simulink model "N3Z_tonetest14b"  (R2014b)
settings: Solver=ode3  SolverMode=SingleTasking  StartTime=0.0  StopTime=1e-4  FixedStep=fpgaclk  RelTol=1e-3
PreLoadFcn:
  | %fpgaclk=1/32.768e6
  | fpgaclk=1/49.162e6
  | 
  | SerialData=[1,zeros(1,11),1,0,0,1]
  | load ../N3workingG/window
  | win=win';  %Go back to using flatter and wider windowed sync function
  | %load ../N3workingG/hanning    %use Hahn window
  | 
  | load ../N3workingG/PREemphasis   %For pre-empasis and deemphasis FIRs
  | 
  | %LUT3=xls2LUT2('../IQI_Qdemod.xls'); LUT3
  | load ../N3workingG/LUT3
  | load ../N3workingG/FIRiq2
  | % xls2LUT
  | 
  | GetProgFiles
  | 
  | PinAssignments    %Get Pin references for TE0722
  | 
  | 
  | 
  | 
  | 
  | %LCD
  | LCDdata=[LCD_D7,LCD_D6,LCD_D5,LCD_D4,LCD_D3,LCD_D2,LCD_D1,LCD_D0] %Note MSB...LSB!
  | LCDctrl=[LCD_E,LCD_RW,LCD_RS];
  | 
  | %for RS232 on pins 3 and 5 of USBB
  | 
  | %BT chip connections for WT12
  | 
  | RX_BT=RXD
  | TX_BT=TXD
  | 
  | RST_BB=RES
  | 
  | %PCMC=PCMC
  | %PCMS=PCMS
  | %PCMI=PCMI
  | %PCMO=PCMO
  | 
  | %Aliases:
  | SRDBT=PCMI
  | STDBT=PCMO
  | SCLK_BT=PCMC
  | SFS_BT=PCMS
  | 
  | %ADC control
  | 
  | %SDOA=SDOA
  | %SDOB=SDOB
  | %SCK=SCK
  | CONV=Csbar
  | CAL=Cal
  | 
  | ADC_G=[ADC_G3,ADC_G2,ADC_G1,ADC_G0]
  | %PD settings hard coded now
  | 
  | %%%%%%
  | TX_LOW=TX_Low
  | ... (+11 lines)
StartFcn:
  | SerialData=[1,zeros(1,11),1,0,0,1]
values from neighbouring files (symbols this model uses):
  ADC_G0 = {'P10'}    [PinAssignments.m]
  ADC_G1 = {'P11'}    [PinAssignments.m]
  ADC_G2 = {'N14'}    [PinAssignments.m]
  ADC_G3 = {'M11'}    [PinAssignments.m]
  Cal = {'L12'}    [PinAssignments.m]
  Csbar = {'M12'}    [PinAssignments.m]
  LCD_D0 = {'J13'}    [PinAssignments.m]
  LCD_D1 = {'J14'}    [PinAssignments.m]
  LCD_D2 = {'F15'}    [PinAssignments.m]
  LCD_D3 = {'H14'}    [PinAssignments.m]
  LCD_D4 = {'G12'}    [PinAssignments.m]
  LCD_D5 = {'L15'}    [PinAssignments.m]
  LCD_D6 = {'M14'}    [PinAssignments.m]
  LCD_D7 = {'K15'}    [PinAssignments.m]
  PCMC = {'H11'}    [PinAssignments.m]
  PCMI = {'H12'}    [PinAssignments.m]
  PCMO = {'N13'}    [PinAssignments.m]
  PCMS = {'M10'}    [PinAssignments.m]
  RES = {'G11'}    [PinAssignments.m]
  RXD = {'H13'}    [PinAssignments.m]
  TX_Low = {'P15'}    [PinAssignments.m]
  TXD = {'P13'}    [PinAssignments.m]
undefined symbols (not defined in the file or in its folder): AXI4, FIRRX, FIRTX, Lite
libraries: xbsIndex_r4 x1214, MyFunctions x43
(part 6 of 9)

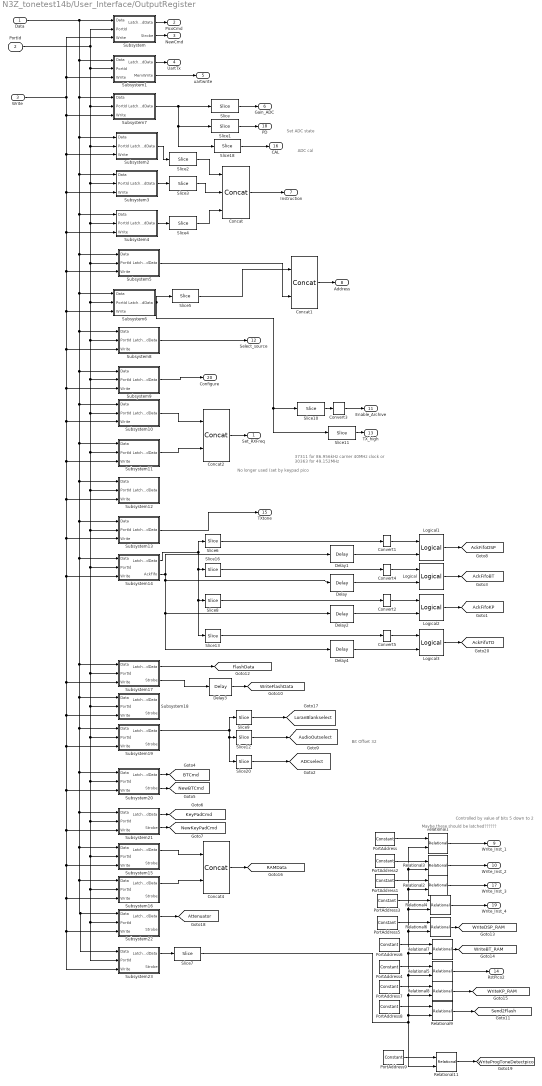
== system N3Z_tonetest14b/User_Interface/OutputRegister ==
  note: No longer used (set by keypad pico
  note: ADC cal
  note: 37311 for 86.956kHz carrier 40MHz clock
      | or 30363 for 49.152MHz
  note: Controlled by value of bits 5 down to 2
  note: Maybe these should be latched??????
  note: Bit Offset 32
  note: Set ADC state
  Data : Inport
  PortId : Inport  Port=2
  Write : Inport  Port=3
  Concat : xbsIndex_r4/Concat  num_inputs=3  dbl_ovrd=off  block_type=concat
      settings: block_version=8.2.02
  Concat1 : xbsIndex_r4/Concat  num_inputs=2  dbl_ovrd=off  block_type=concat
      settings: block_version=8.2.02
  Concat2 : xbsIndex_r4/Concat  num_inputs=2  dbl_ovrd=off  block_type=concat
      settings: block_version=8.2.02
  Concat4 : xbsIndex_r4/Concat  num_inputs=2  dbl_ovrd=off  block_type=concat
      settings: block_version=8.2.02
  Convert{1..5} (5 alike) : xbsIndex_r4/Convert  gui_display_data_type=Fixed-point  arith_type=Boolean  n_bits=16  bin_pt=0  float_type=Single  exp_bits=8  fraction_bits=24  quantization=Truncate  overflow=Wrap  en=off  latency=0  pipeline=off  dbl_ovrd=off  block_type=convert
      settings: xl_area=[0, 0, 0, 0, 0, 0, 0]  block_version=VER_STRING_GOES_HERE
  Delay{,1..4} (5 alike) : xbsIndex_r4/Delay  rst=off  infoeditControl=Selection of Reset will increase slice count due to use of real FFs and instead of SRLs  en=off  latency=1  reg_retiming=off  dbl_ovrd=off  block_type=delay
      settings: infoedit=Hardware notes: A delay line is a chain, each link of which is an SRL16 followed by a flip-flop. If register retiming is enabled, the delay line is a chain of flip-flops.  block_version=8.2.02
  Logical{,1..3} (4 alike) : xbsIndex_r4/Logical  logical_function=AND  inputs=2  en=off  latency=0  precision=Full  arith_type=Unsigned  n_bits=16  bin_pt=0  align_bp=on  dbl_ovrd=off  block_type=logical
      settings: block_version=8.2.02
  PortAddress : xbsIndex_r4/Constant  const=1  gui_display_data_type=Fixed-point  arith_type=Unsigned  n_bits=4  bin_pt=0  preci_type=Single  exp_width=8  frac_width=24  explicit_period=on  period=fpgaclk  equ=P=C  opselect=C  inp2=PCIN>>17  opr=+  inp1=P  carry=CIN  dbl_ovrd=off  block_type=constant
      settings: block_version=VER_STRING_GOES_HERE
  PortAddress1 : xbsIndex_r4/Constant  const=3  gui_display_data_type=Fixed-point  arith_type=Unsigned  n_bits=4  bin_pt=0  preci_type=Single  exp_width=8  frac_width=24  explicit_period=on  period=fpgaclk  equ=P=C  opselect=C  inp2=PCIN>>17  opr=+  inp1=P  carry=CIN  dbl_ovrd=off  block_type=constant
      settings: block_version=VER_STRING_GOES_HERE
  PortAddress2 : xbsIndex_r4/Constant  const=2  gui_display_data_type=Fixed-point  arith_type=Unsigned  n_bits=4  bin_pt=0  preci_type=Single  exp_width=8  frac_width=24  explicit_period=on  period=fpgaclk  equ=P=C  opselect=C  inp2=PCIN>>17  opr=+  inp1=P  carry=CIN  dbl_ovrd=off  block_type=constant
      settings: block_version=VER_STRING_GOES_HERE
  PortAddress3 : xbsIndex_r4/Constant  const=4  gui_display_data_type=Fixed-point  arith_type=Unsigned  n_bits=4  bin_pt=0  preci_type=Single  exp_width=8  frac_width=24  explicit_period=on  period=fpgaclk  equ=P=C  opselect=C  inp2=PCIN>>17  opr=+  inp1=P  carry=CIN  dbl_ovrd=off  block_type=constant
      settings: block_version=VER_STRING_GOES_HERE
  PortAddress4 : xbsIndex_r4/Constant  const=7  gui_display_data_type=Fixed-point  arith_type=Unsigned  n_bits=4  bin_pt=0  preci_type=Single  exp_width=8  frac_width=24  explicit_period=on  period=fpgaclk  equ=P=C  opselect=C  inp2=PCIN>>17  opr=+  inp1=P  carry=CIN  dbl_ovrd=off  block_type=constant
      settings: block_version=VER_STRING_GOES_HERE
  PortAddress5 : xbsIndex_r4/Constant  const=5  gui_display_data_type=Fixed-point  arith_type=Unsigned  n_bits=4  bin_pt=0  preci_type=Single  exp_width=8  frac_width=24  explicit_period=on  period=fpgaclk  equ=P=C  opselect=C  inp2=PCIN>>17  opr=+  inp1=P  carry=CIN  dbl_ovrd=off  block_type=constant
      settings: block_version=VER_STRING_GOES_HERE
  PortAddress6 : xbsIndex_r4/Constant  const=6  gui_display_data_type=Fixed-point  arith_type=Unsigned  n_bits=4  bin_pt=0  preci_type=Single  exp_width=8  frac_width=24  explicit_period=on  period=fpgaclk  equ=P=C  opselect=C  inp2=PCIN>>17  opr=+  inp1=P  carry=CIN  dbl_ovrd=off  block_type=constant
      settings: block_version=VER_STRING_GOES_HERE
  PortAddress7 : xbsIndex_r4/Constant  const=8  gui_display_data_type=Fixed-point  arith_type=Unsigned  n_bits=4  bin_pt=0  preci_type=Single  exp_width=8  frac_width=24  explicit_period=on  period=fpgaclk  equ=P=C  opselect=C  inp2=PCIN>>17  opr=+  inp1=P  carry=CIN  dbl_ovrd=off  block_type=constant
      settings: block_version=VER_STRING_GOES_HERE
  PortAddress8 : xbsIndex_r4/Constant  const=9  gui_display_data_type=Fixed-point  arith_type=Unsigned  n_bits=4  bin_pt=0  preci_type=Single  exp_width=8  frac_width=24  explicit_period=on  period=fpgaclk  equ=P=C  opselect=C  inp2=PCIN>>17  opr=+  inp1=P  carry=CIN  dbl_ovrd=off  block_type=constant
      settings: block_version=VER_STRING_GOES_HERE
  PortAddress9 : xbsIndex_r4/Constant  const=10  gui_display_data_type=Fixed-point  arith_type=Unsigned  n_bits=4  bin_pt=0  preci_type=Single  exp_width=8  frac_width=24  explicit_period=on  period=fpgaclk  equ=P=C  opselect=C  inp2=PCIN>>17  opr=+  inp1=P  carry=CIN  dbl_ovrd=off  block_type=constant
      settings: block_version=VER_STRING_GOES_HERE
  Relational{1..9,11} (10 alike) : xbsIndex_r4/Relational  mode=a=b  op_type=Bool  en=off  latency=1  dbl_ovrd=off  block_type=relational
      settings: xl_area=[2 0 0 4 0 0 0]  block_version=VER_STRING_GOES_HERE
  Slice : xbsIndex_r4/Slice  nbits=4  boolean_output=off  mode=Lower Bit Location + Width  bit1=0  base1=MSB of Input  bit0=0  base0=LSB of Input  dbl_ovrd=off  block_type=slice
      settings: block_version=8.2.02
  Slice1 : xbsIndex_r4/Slice  nbits=3  boolean_output=off  mode=Lower Bit Location + Width  bit1=0  base1=MSB of Input  bit0=4  base0=LSB of Input  dbl_ovrd=off  block_type=slice
      settings: block_version=8.2.02
  Slice{8,10,13,20} (4 alike) : xbsIndex_r4/Slice  nbits=1  boolean_output=off  mode=Lower Bit Location + Width  bit1=3  base1=MSB of Input  bit0=6  base0=LSB of Input  dbl_ovrd=off  block_type=slice
      settings: block_version=8.2.02
  Slice11 : xbsIndex_r4/Slice  nbits=1  boolean_output=off  mode=Lower Bit Location + Width  bit1=3  base1=MSB of Input  bit0=7  base0=LSB of Input  dbl_ovrd=off  block_type=slice
      settings: block_version=8.2.02
  Slice12 : xbsIndex_r4/Slice  nbits=1  boolean_output=off  mode=Lower Bit Location + Width  bit1=3  base1=MSB of Input  bit0=5  base0=LSB of Input  dbl_ovrd=off  block_type=slice
      settings: block_version=8.2.02
  Slice16 : xbsIndex_r4/Slice  nbits=1  boolean_output=off  mode=Lower Bit Location + Width  bit1=3  base1=MSB of Input  bit0=5  base0=LSB of Input  dbl_ovrd=off  block_type=slice
      settings: block_version=8.2.02
  Slice18 : xbsIndex_r4/Slice  nbits=1  boolean_output=off  mode=Lower Bit Location + Width  bit1=0  base1=MSB of Input  bit0=7  base0=LSB of Input  dbl_ovrd=off  block_type=slice
      settings: block_version=8.2.02
  Slice2 : xbsIndex_r4/Slice  nbits=6  boolean_output=off  mode=Lower Bit Location + Width  bit1=3  base1=MSB of Input  bit0=0  base0=LSB of Input  dbl_ovrd=off  block_type=slice
      settings: infoedit="Extracts a given range of bits from each input sample and presents it at the output.  The output type is ordinarily unsigned with binary point at zero, but can be Boolean when the slice is one bit wide.<P><P>Hardware notes: In hardware this block costs nothing."  block_version=8.2.02
  Slice3 : xbsIndex_r4/Slice  nbits=6  boolean_output=off  mode=Lower Bit Location + Width  bit1=3  base1=MSB of Input  bit0=0  base0=LSB of Input  dbl_ovrd=off  block_type=slice
      settings: infoedit="Extracts a given range of bits from each input sample and presents it at the output.  The output type is ordinarily unsigned with binary point at zero, but can be Boolean when the slice is one bit wide.<P><P>Hardware notes: In hardware this block costs nothing."  block_version=8.2.02
  Slice4 : xbsIndex_r4/Slice  nbits=6  boolean_output=off  mode=Lower Bit Location + Width  bit1=3  base1=MSB of Input  bit0=0  base0=LSB of Input  dbl_ovrd=off  block_type=slice
      settings: infoedit="Extracts a given range of bits from each input sample and presents it at the output.  The output type is ordinarily unsigned with binary point at zero, but can be Boolean when the slice is one bit wide.<P><P>Hardware notes: In hardware this block costs nothing."  block_version=8.2.02
  Slice5 : xbsIndex_r4/Slice  nbits=3  boolean_output=off  mode=Lower Bit Location + Width  bit1=3  base1=MSB of Input  bit0=0  base0=LSB of Input  dbl_ovrd=off  block_type=slice
      settings: block_version=8.2.02
  Slice6 : xbsIndex_r4/Slice  nbits=1  boolean_output=off  mode=Lower Bit Location + Width  bit1=3  base1=MSB of Input  bit0=4  base0=LSB of Input  dbl_ovrd=off  block_type=slice
      settings: block_version=8.2.02
  Slice7 : xbsIndex_r4/Slice  nbits=4  boolean_output=off  mode=Lower Bit Location + Width  bit1=3  base1=MSB of Input  bit0=2  base0=LSB of Input  dbl_ovrd=off  block_type=slice
      settings: block_version=8.2.02
  Slice9 : xbsIndex_r4/Slice  nbits=1  boolean_output=off  mode=Lower Bit Location + Width  bit1=3  base1=MSB of Input  bit0=4  base0=LSB of Input  dbl_ovrd=off  block_type=slice
      settings: block_version=8.2.02
  Subsystem : Subsystem
  Subsystem1 : Subsystem
  Subsystem10 : Subsystem
  Subsystem11 : Subsystem
  Subsystem12 : Subsystem
  Subsystem13 : Subsystem
  Subsystem14 : Subsystem
  Subsystem15 : Subsystem
  Subsystem16 : Subsystem
  Subsystem17 : Subsystem
  Subsystem18 : Subsystem
  Subsystem19 : Subsystem
  Subsystem2 : Subsystem
  Subsystem20 : Subsystem
  Subsystem21 : Subsystem
  Subsystem22 : Subsystem
  Subsystem23 : Subsystem
  Subsystem3 : Subsystem
  Subsystem4 : Subsystem
  Subsystem5 : Subsystem
  Subsystem6 : Subsystem
  Subsystem7 : Subsystem
  Subsystem8 : Subsystem
  Subsystem9 : Subsystem
  Set_RXFreq : Outport
  PicoCmd : Outport  Port=2
  NewCmd : Outport  Port=3
  UartTx : Outport  Port=4
  uartwrite : Outport  Port=5
  Gain_ADC : Outport  Port=6
  Instruction : Outport  Port=7
  Address : Outport  Port=8
  Write_Inst_1 : Outport  Port=9
  Write_Inst_2 : Outport  Port=10
  Enable_Archive : Outport  Port=11
  Select_source : Outport  Port=12
  TX_high : Outport  Port=13
  RstPico2 : Outport  Port=14
  TXtone : Outport  Port=15
  CAL : Outport  Port=16
  Write_Inst_3 : Outport  Port=17
  PD : Outport  Port=18
  Write_Inst_4 : Outport  Port=19
  Configure : Outport  Port=20
  tag scope: ADCselect=global, AckFifoBT=global, AckFifoDSP=global, AckFifoKP=global, AckFifoTD=global, Attenuator=global, AudioOutselect=global, BTCmd=global, FlashData=global, KeyPadCmd=global, LoranBlankselect=global, NewBTCmd=global, NewKeyPadCmd=global, RAMData=global, Send2Flash=global, WriteBT_RAM=global, WriteDSP_RAM=global, WriteFlashData=global, WriteKP_RAM=global, WriteProgToneDetectpico=global
  wires:
  PortId/1 -> Subsystem/2(PortId), Subsystem1/2(PortId), Subsystem7/2(PortId), Subsystem2/2(PortId), Subsystem3/2(PortId), Subsystem4/2(PortId), Subsystem5/2(PortId), Subsystem6/2(PortId), Subsystem8/2(PortId), Subsystem9/2(PortId), Subsystem10/2(PortId), Subsystem11/2(PortId), Subsystem12/2(PortId), Subsystem13/2(PortId), Subsystem14/2(PortId), Subsystem17/2(PortId), Subsystem18/2(PortId), Subsystem19/2(PortId), Subsystem20/2(PortId), Subsystem21/2(PortId), Subsystem15/2(PortId), Subsystem16/2(PortId), Subsystem23/2(PortId), Subsystem22/2(PortId)
  Data/1 -> Subsystem/1(Data), Subsystem1/1(Data), Subsystem7/1(Data), Subsystem2/1(Data), Subsystem3/1(Data), Subsystem4/1(Data), Subsystem5/1(Data), Subsystem6/1(Data), Subsystem8/1(Data), Subsystem9/1(Data), Subsystem10/1(Data), Subsystem11/1(Data), Subsystem12/1(Data), Subsystem13/1(Data), Subsystem14/1(Data), Subsystem17/1(Data), Subsystem18/1(Data), Subsystem19/1(Data), Subsystem20/1(Data), Subsystem21/1(Data), Subsystem15/1(Data), Subsystem16/1(Data), Subsystem23/1(Data), Subsystem22/1(Data)
  Subsystem1/1(LatchedData) -> UartTx/1
  Write/1 -> Subsystem1/3(Write), Subsystem/3(Write), Subsystem7/3(Write), Subsystem2/3(Write), Subsystem3/3(Write), Subsystem4/3(Write), Subsystem5/3(Write), Subsystem6/3(Write), Subsystem8/3(Write), Subsystem9/3(Write), Subsystem10/3(Write), Subsystem11/3(Write), Subsystem12/3(Write), Subsystem13/3(Write), Subsystem14/3(Write), Subsystem17/3(Write), Subsystem18/3(Write), Subsystem19/3(Write), Subsystem20/3(Write), Subsystem21/3(Write), Subsystem15/3(Write), Subsystem16/3(Write), Subsystem23/3(Write), Subsystem22/3(Write)
  Subsystem7/1(LatchedData) -> Slice/1, Slice1/1, Slice18/1
  Subsystem/1(LatchedData) -> PicoCmd/1
  Subsystem1/2(MemWrite) -> uartwrite/1
  Slice/1 -> Gain_ADC/1
  Subsystem2/1(LatchedData) -> Slice2/1
  Subsystem3/1(LatchedData) -> Slice3/1
  Subsystem4/1(LatchedData) -> Slice4/1
  Slice2/1 -> Concat/1
  Slice3/1 -> Concat/2
  Slice4/1 -> Concat/3
  Concat/1 -> Instruction/1
  Subsystem6/1(LatchedData) -> Slice5/1, Slice10/1, Slice11/1
  Concat1/1 -> Address/1
  Subsystem10/1(LatchedData) -> Concat2/1
  Subsystem11/1(LatchedData) -> Concat2/2
  Concat2/1 -> Set_RXFreq/1
  Slice5/1 -> Concat1/1
  Subsystem5/1(LatchedData) -> Concat1/2
  Convert3/1 -> Enable_Archive/1
  Slice11/1 -> TX_high/1
  Subsystem/2(Strobe) -> NewCmd/1
  Subsystem13/1(LatchedData) -> TXtone/1
  Delay/1 -> Logical/2
  Slice16/1 -> Convert4/1
  Convert4/1 -> Logical/1
  Subsystem19/1(LatchedData) -> Slice20/1, Slice12/1, Slice9/1
  Slice18/1 -> CAL/1
  Slice20/1 -> [ADCselect]
  PortAddress/1 -> Relational1/1
  Slice7/1 -> Relational11/2, Relational4/2, Relational1/2, Relational3/2, Relational2/2, Relational6/2, Relational7/2, Relational5/2, Relational8/2, Relational9/2
  Relational1/1 -> Write_Inst_1/1
  PortAddress1/1 -> Relational2/1
  Relational2/1 -> Write_Inst_3/1
  PortAddress2/1 -> Relational3/1
  Relational3/1 -> Write_Inst_2/1
  PortAddress3/1 -> Relational4/1
  Relational4/1 -> Write_Inst_4/1
  PortAddress4/1 -> Relational5/1
  Relational5/1 -> RstPico2/1
  Subsystem20/1(LatchedData) -> [BTCmd]
  Subsystem20/2(Strobe) -> [NewBTCmd]
  Subsystem21/1(LatchedData) -> [KeyPadCmd]
  Subsystem21/2(Strobe) -> [NewKeyPadCmd]
  Subsystem8/1(LatchedData) -> Select_source/1
  Delay1/1 -> Logical1/2
  Slice6/1 -> Convert1/1
  Convert1/1 -> Logical1/1
  Delay2/1 -> Logical2/2
  Slice8/1 -> Convert2/1
  Convert2/1 -> Logical2/1
  Logical1/1 -> [AckFifoDSP]
  Logical/1 -> [AckFifoBT]
  Logical2/1 -> [AckFifoKP]
  Slice12/1 -> [AudioOutselect]
  Slice1/1 -> PD/1
  Slice10/1 -> Convert3/1
  PortAddress5/1 -> Relational6/1
  Relational6/1 -> [WriteDSP_RAM]
  PortAddress6/1 -> Relational7/1
  Relational7/1 -> [WriteBT_RAM]
  Delay3/1 -> [WriteFlashData]
  Subsystem17/1(LatchedData) -> [FlashData]
  Subsystem17/2(Strobe) -> Delay3/1
  PortAddress7/1 -> Relational8/1
  Relational8/1 -> [WriteKP_RAM]
  PortAddress8/1 -> Relational9/1
  Relational9/1 -> [Send2Flash]
  Subsystem15/1(LatchedData) -> Concat4/1
  Subsystem16/1(LatchedData) -> Concat4/2
  Concat4/1 -> [RAMData]
  Slice9/1 -> [LoranBlankselect]
  Subsystem22/1(LatchedData) -> [Attenuator]
  Subsystem23/1(LatchedData) -> Slice7/1
  Subsystem9/1(LatchedData) -> Configure/1
  PortAddress9/1 -> Relational11/1
  Relational11/1 -> [WriteProgToneDetectpico]
  Subsystem14/1(LatchedData) -> Slice6/1, Slice16/1, Slice13/1, Slice8/1
  Subsystem14/2(AckFifo) -> Delay1/1, Delay/1, Delay4/1, Delay2/1
  Delay4/1 -> Logical3/2
  Slice13/1 -> Convert5/1
  Convert5/1 -> Logical3/1
  Logical3/1 -> [AckFifoTD]

== system N3Z_tonetest14b/User_Interface/Subsystem1 ==
  note: Enable on address 0
  PortId : Inport
  rs : Inport  Port=2
  Convert : xbsIndex_r4/Convert  gui_display_data_type=Fixed-point  arith_type=Unsigned  n_bits=1  bin_pt=0  float_type=Single  exp_bits=8  fraction_bits=24  quantization=Truncate  overflow=Wrap  en=off  latency=0  pipeline=off  dbl_ovrd=off  block_type=convert
      settings: block_version=VER_STRING_GOES_HERE
  Logical : xbsIndex_r4/Logical  logical_function=AND  inputs=2  en=off  latency=0  precision=Full  arith_type=Unsigned  n_bits=16  bin_pt=0  align_bp=on  dbl_ovrd=off  block_type=logical
      settings: block_version=VER_STRING_GOES_HERE
  Logical1 : xbsIndex_r4/Logical  logical_function=NOR  inputs=4  en=off  latency=1  precision=Full  arith_type=Unsigned  n_bits=16  bin_pt=0  align_bp=on  dbl_ovrd=off  block_type=logical
      settings: block_version=VER_STRING_GOES_HERE
  Register : xbsIndex_r4/Register  init=0  rst=off  en=off  dbl_ovrd=off  block_type=register
      settings: block_version=VER_STRING_GOES_HERE
  Slice : xbsIndex_r4/Slice  nbits=1  boolean_output=off  mode=Lower Bit Location + Width  bit1=0  base1=MSB of Input  bit0=0  base0=LSB of Input  dbl_ovrd=off  block_type=slice
      settings: block_version=VER_STRING_GOES_HERE
  Slice1 : xbsIndex_r4/Slice  nbits=1  boolean_output=off  mode=Lower Bit Location + Width  bit1=0  base1=MSB of Input  bit0=1  base0=LSB of Input  dbl_ovrd=off  block_type=slice
      settings: block_version=VER_STRING_GOES_HERE
  Slice2 : xbsIndex_r4/Slice  nbits=1  boolean_output=off  mode=Lower Bit Location + Width  bit1=0  base1=MSB of Input  bit0=2  base0=LSB of Input  dbl_ovrd=off  block_type=slice
      settings: block_version=VER_STRING_GOES_HERE
  Slice3 : xbsIndex_r4/Slice  nbits=1  boolean_output=off  mode=Lower Bit Location + Width  bit1=0  base1=MSB of Input  bit0=3  base0=LSB of Input  dbl_ovrd=off  block_type=slice
      settings: block_version=VER_STRING_GOES_HERE
  read_buffer : Outport
  wires:
  Register/1 -> Convert/1
  Logical1/1 -> Logical/1
  Convert/1 -> Logical/2
  PortId/1 -> Slice/1, Slice1/1, Slice2/1, Slice3/1
  Logical/1 -> read_buffer/1
  rs/1 -> Register/1
  Slice/1 -> Logical1/1
  Slice1/1 -> Logical1/2
  Slice2/1 -> Logical1/3
  Slice3/1 -> Logical1/4

== system N3Z_tonetest14b/ADCRead/Subsystem1/SCKgenerator ==
  Trig : Inport
  Constant : xbsIndex_r4/Constant  const=1  gui_display_data_type=Boolean  arith_type=Boolean  n_bits=1  bin_pt=0  preci_type=Single  exp_width=8  frac_width=24  explicit_period=on  period=fpgaclk  equ=P=C  opselect=C  inp2=PCIN>>17  opr=+  inp1=P  carry=CIN  dbl_ovrd=off  block_type=constant
      settings: block_version=VER_STRING_GOES_HERE
  Constant1 : xbsIndex_r4/Constant  const=19  gui_display_data_type=Fixed-point  arith_type=Unsigned  n_bits=5  bin_pt=0  preci_type=Single  exp_width=8  frac_width=24  explicit_period=on  period=fpgaclk  equ=P=C  opselect=C  inp2=PCIN>>17  opr=+  inp1=P  carry=CIN  dbl_ovrd=off  block_type=constant
      settings: block_version=VER_STRING_GOES_HERE
  Convert1 : xbsIndex_r4/Convert  gui_display_data_type=Fixed-point  arith_type=Boolean  n_bits=8  bin_pt=6  float_type=Single  exp_bits=8  fraction_bits=24  quantization=Truncate  overflow=Wrap  en=off  latency=0  pipeline=off  dbl_ovrd=off  block_type=convert
      settings: xl_area=[0 0 0 0 0 0 0]  block_version=VER_STRING_GOES_HERE
  Convert2 : xbsIndex_r4/Convert  gui_display_data_type=Fixed-point  arith_type=Boolean  n_bits=8  bin_pt=6  float_type=Single  exp_bits=8  fraction_bits=24  quantization=Truncate  overflow=Wrap  en=off  latency=0  pipeline=off  dbl_ovrd=off  block_type=convert
      settings: xl_area=[0 0 0 0 0 0 0]  block_version=VER_STRING_GOES_HERE
  Counter : xbsIndex_r4/Counter  cnt_type=Count Limited  cnt_to=Inf  operation=Up  start_count=0  cnt_by_val=1  arith_type=Unsigned  n_bits=6  bin_pt=0  load_pin=off  rst=on  en=on  explicit_period=on  period=fpgaclk  use_behavioral_HDL=off  implementation=Fabric  use_rpm=on  dbl_ovrd=off  block_type=counter
      settings: xl_area=[3 4 0 5 0 0 0]  block_version=VER_STRING_GOES_HERE
  Counter1 : xbsIndex_r4/Counter  cnt_type=Count Limited  cnt_to=Inf  operation=Up  start_count=0  cnt_by_val=1  arith_type=Unsigned  n_bits=1  bin_pt=0  load_pin=off  rst=on  en=on  explicit_period=on  period=fpgaclk  use_behavioral_HDL=off  implementation=Fabric  use_rpm=on  dbl_ovrd=off  block_type=counter
      settings: xl_area=[3 3 0 4 0 0 0]  block_version=VER_STRING_GOES_HERE
  Delay2 : xbsIndex_r4/Delay  rst=off  infoeditControl=Selection of Reset will increase slice count due to use of real FFs and instead of SRLs  en=off  latency=1  reg_retiming=off  dbl_ovrd=off  block_type=delay
      settings: infoedit=Hardware notes: A delay line is a chain, each link of which is an SRL16 followed by a flip-flop. If register retiming is enabled, the delay line is a chain of flip-flops.  xl_area=[1 1 0 0 0 0 0]  block_version=VER_STRING_GOES_HERE
  Inverter : xbsIndex_r4/Inverter  en=off  latency=0  dbl_ovrd=off  block_type=inv
      settings: xl_area=[0 0 0 0 0 0 0]  block_version=VER_STRING_GOES_HERE
  Monostable1 : MyFunctions/Monostable
      link override Delay1: xl_area=[1 1 0 0 0 0 0]
      link override Inverter: xl_area=[0 0 0 0 0 0 0]
      link override Logical: xl_area=[1 0 0 1 0 0 0]
  Monostable2 : MyFunctions/Monostable
      link override Delay1: xl_area=[1 1 0 0 0 0 0]
      link override Inverter: xl_area=[0 0 0 0 0 0 0]
      link override Logical: xl_area=[1 0 0 1 0 0 0]
  Register3 : xbsIndex_r4/Register  init=0  rst=on  en=on  dbl_ovrd=off  block_type=register
      settings: xl_area=[1 1 0 0 0 0 0]  block_version=VER_STRING_GOES_HERE
  Relational : xbsIndex_r4/Relational  mode=a>=b  op_type=Bool  en=off  latency=1  dbl_ovrd=off  block_type=relational
      settings: block_version=9.2.01
  Slice1 : xbsIndex_r4/Slice  nbits=1  boolean_output=off  mode=Upper Bit Location + Width  bit1=0  base1=MSB of Input  bit0=0  base0=LSB of Input  dbl_ovrd=off  block_type=slice
      settings: infoedit="Extracts a given range of bits from each input sample and presents it at the output.  The output type is ordinarily unsigned with binary point at zero, but can be Boolean when the slice is one bit wide.<P><P>Hardware notes: In hardware this block costs nothing."  block_version=VER_STRING_GOES_HERE
  Slice2 : xbsIndex_r4/Slice  nbits=1  boolean_output=off  mode=Upper Bit Location + Width  bit1=0  base1=MSB of Input  bit0=0  base0=LSB of Input  dbl_ovrd=off  block_type=slice
      settings: infoedit="Extracts a given range of bits from each input sample and presents it at the output.  The output type is ordinarily unsigned with binary point at zero, but can be Boolean when the slice is one bit wide.<P><P>Hardware notes: In hardware this block costs nothing."  block_version=VER_STRING_GOES_HERE
  DataReady : Outport
  SCK : Outport  Port=2
  Conv : Outport  Port=3
  DataValid : Outport  Port=4
  wires:
  Constant/1 -> Register3/1
  Monostable1/1 -> Register3/2, Counter1/1
  Register3/1 -> Counter/1, Conv/1, Inverter/1
  Counter/1 -> Slice2/1, Relational/1
  Delay2/1 -> Monostable2/1
  Monostable2/1 -> Register3/3, DataReady/1
  Inverter/1 -> Counter1/2
  Counter1/1 -> Slice1/1
  Slice1/1 -> Convert2/1
  Convert2/1 -> Counter/2, SCK/1
  Trig/1 -> Monostable1/1
  Slice2/1 -> Convert1/1
  Convert1/1 -> Delay2/1
  Constant1/1 -> Relational/2
  Relational/1 -> DataValid/1

== system N3Z_tonetest14b/DSProcessor1/OutputRegister/LevelMonitor ==
  note: Use 10 bt signed input
  note: Pulses at 8kHz
  note: reset at ~0.5Hz - so divide 8kHz by 2^14
  note: 19 bits should be fairly conservative
  In1 : Inport
  En : Inport  Port=2
  AddSub : xbsIndex_r4/AddSub  mode=Addition or Subtraction  use_carryin=off  use_carryout=off  en=on  latency=1  precision=User Defined  arith_type=Unsigned  n_bits=19+1+4+2  bin_pt=0  quantization=Truncate  overflow=Saturate  use_behavioral_HDL=off  hw_selection=Fabric  pipelined=off  dbl_ovrd=off  block_type=addsub
      settings: block_version=12.2
  Convert : xbsIndex_r4/Convert  gui_display_data_type=Boolean  arith_type=Boolean  n_bits=16  bin_pt=14  float_type=Single  exp_bits=8  fraction_bits=24  quantization=Truncate  overflow=Wrap  en=off  latency=0  pipeline=off  dbl_ovrd=off  block_type=convert
      settings: block_version=12.2
  Convert1 : xbsIndex_r4/Convert  gui_display_data_type=Fixed-point  arith_type=Boolean  n_bits=16  bin_pt=14  float_type=Single  exp_bits=8  fraction_bits=24  quantization=Truncate  overflow=Wrap  en=off  latency=0  pipeline=off  dbl_ovrd=off  block_type=convert
      settings: block_version=12.2
  Convert2 : xbsIndex_r4/Convert  gui_display_data_type=Fixed-point  arith_type="Signed  (2's comp)"  n_bits=10  bin_pt=0  float_type=Single  exp_bits=8  fraction_bits=24  quantization=Truncate  overflow=Wrap  en=off  latency=0  pipeline=off  dbl_ovrd=off  block_type=convert
      settings: block_version=12.2
  Counter : xbsIndex_r4/Counter  cnt_type=Free Running  cnt_to=Inf  operation=Up  start_count=0  cnt_by_val=1  arith_type=Unsigned  n_bits=11+4  bin_pt=0  load_pin=off  rst=off  en=on  explicit_period=on  period=fpgaclk  use_behavioral_HDL=off  implementation=Fabric  dbl_ovrd=off  block_type=counter
      settings: block_version=12.2
  Delay : xbsIndex_r4/Delay  rst=off  infoeditControl=Selection of Reset will increase slice count due to use of real FFs and instead of SRLs  en=off  latency=2  reg_retiming=off  dbl_ovrd=off  block_type=delay
  Delay1 : xbsIndex_r4/Delay  rst=off  infoeditControl=Selection of Reset will increase slice count due to use of real FFs and instead of SRLs  en=off  latency=2  reg_retiming=off  dbl_ovrd=off  block_type=delay
  Monostable : MyFunctions/Monostable
  Monostable2 : MyFunctions/Monostable
  Register : xbsIndex_r4/Register  init=0  rst=on  en=on  dbl_ovrd=off  block_type=register
      settings: block_version=12.2
  Register1 : xbsIndex_r4/Register  init=0  rst=off  en=on  dbl_ovrd=off  block_type=register
      settings: block_version=12.2
  Slice1 : xbsIndex_r4/Slice  nbits=1  boolean_output=off  mode=Upper Bit Location + Width  bit1=0  base1=MSB of Input  bit0=0  base0=LSB of Input  dbl_ovrd=off  block_type=slice
      settings: block_version=12.2
  Slice2 : xbsIndex_r4/Slice  nbits=1  boolean_output=off  mode=Upper Bit Location + Width  bit1=0  base1=MSB of Input  bit0=0  base0=LSB of Input  dbl_ovrd=off  block_type=slice
      settings: block_version=12.2
  Slice3 : xbsIndex_r4/Slice  nbits=16  boolean_output=off  mode=Upper Bit Location + Width  bit1=0  base1=MSB of Input  bit0=0  base0=LSB of Input  dbl_ovrd=off  block_type=slice
      settings: block_version=12.2
  Slice4 : xbsIndex_r4/Slice  nbits=10  boolean_output=off  mode=Upper Bit Location + Width  bit1=0  base1=MSB of Input  bit0=0  base0=LSB of Input  dbl_ovrd=off  block_type=slice
      settings: block_version=12.2
  SignalLevel : Outport
  wires:
  In1/1 -> Slice1/1, Slice4/1
  AddSub/1 -> Register/1
  En/1 -> Monostable2/1
  Slice1/1 -> Convert/1
  Convert/1 -> AddSub/3
  Register/1 -> AddSub/1, Slice3/1
  Counter/1 -> Slice2/1
  Monostable/1 -> Convert1/1
  Convert1/1 -> Register1/2, Delay1/1
  Slice2/1 -> Monostable/1
  Slice3/1 -> Register1/1
  Slice4/1 -> Convert2/1
  Convert2/1 -> AddSub/2
  Monostable2/1 -> Counter/1, AddSub/4, Delay/1
  Register1/1 -> SignalLevel/1
  Delay/1 -> Register/3
  Delay1/1 -> Register/2

== system N3Z_tonetest14b/DSProcessor1/OutputRegister/LevelMonitor1 ==
  note: Use 10 bt signed input
  note: Pulses at 8kHz
  note: reset at ~10Hz - so divide 8kHz by 2^10
  note: 18 bits should be fairly conservative - always adding as amp is positive number
  In1 : Inport
  En : Inport  Port=2
  AddSub : xbsIndex_r4/AddSub  mode=Addition  use_carryin=off  use_carryout=off  en=on  latency=1  precision=User Defined  arith_type=Unsigned  n_bits=18+1+4  bin_pt=0  quantization=Truncate  overflow=Saturate  use_behavioral_HDL=off  hw_selection=Fabric  pipelined=off  dbl_ovrd=off  block_type=addsub
      settings: block_version=12.2
  Convert1 : xbsIndex_r4/Convert  gui_display_data_type=Fixed-point  arith_type=Boolean  n_bits=16  bin_pt=14  float_type=Single  exp_bits=8  fraction_bits=24  quantization=Truncate  overflow=Wrap  en=off  latency=0  pipeline=off  dbl_ovrd=off  block_type=convert
      settings: block_version=12.2
  Convert2 : xbsIndex_r4/Convert  gui_display_data_type=Fixed-point  arith_type="Signed  (2's comp)"  n_bits=8  bin_pt=0  float_type=Single  exp_bits=8  fraction_bits=24  quantization=Truncate  overflow=Wrap  en=off  latency=0  pipeline=off  dbl_ovrd=off  block_type=convert
      settings: block_version=12.2
  Counter : xbsIndex_r4/Counter  cnt_type=Free Running  cnt_to=Inf  operation=Up  start_count=0  cnt_by_val=1  arith_type=Unsigned  n_bits=11+4  bin_pt=0  load_pin=off  rst=off  en=on  explicit_period=on  period=fpgaclk  use_behavioral_HDL=off  implementation=Fabric  dbl_ovrd=off  block_type=counter
      settings: block_version=12.2
  Delay : xbsIndex_r4/Delay  rst=off  infoeditControl=Selection of Reset will increase slice count due to use of real FFs and instead of SRLs  en=off  latency=2  reg_retiming=off  dbl_ovrd=off  block_type=delay
  Delay1 : xbsIndex_r4/Delay  rst=off  infoeditControl=Selection of Reset will increase slice count due to use of real FFs and instead of SRLs  en=off  latency=2  reg_retiming=off  dbl_ovrd=off  block_type=delay
  Monostable : MyFunctions/Monostable
  Monostable2 : MyFunctions/Monostable
  Register : xbsIndex_r4/Register  init=0  rst=on  en=on  dbl_ovrd=off  block_type=register
      settings: block_version=12.2
  Register1 : xbsIndex_r4/Register  init=0  rst=off  en=on  dbl_ovrd=off  block_type=register
      settings: block_version=12.2
  Slice2 : xbsIndex_r4/Slice  nbits=1  boolean_output=off  mode=Upper Bit Location + Width  bit1=0  base1=MSB of Input  bit0=0  base0=LSB of Input  dbl_ovrd=off  block_type=slice
      settings: block_version=12.2
  Slice3 : xbsIndex_r4/Slice  nbits=16  boolean_output=off  mode=Upper Bit Location + Width  bit1=0  base1=MSB of Input  bit0=0  base0=LSB of Input  dbl_ovrd=off  block_type=slice
      settings: block_version=12.2
  Slice4 : xbsIndex_r4/Slice  nbits=8  boolean_output=off  mode=Upper Bit Location + Width  bit1=0  base1=MSB of Input  bit0=0  base0=LSB of Input  dbl_ovrd=off  block_type=slice
      settings: block_version=12.2
  SignalLevel : Outport
  wires:
  In1/1 -> Slice4/1
  AddSub/1 -> Register/1
  En/1 -> Monostable2/1
  Register/1 -> AddSub/1, Slice3/1
  Counter/1 -> Slice2/1
  Monostable/1 -> Convert1/1
  Convert1/1 -> Register1/2, Delay1/1
  Slice2/1 -> Monostable/1
  Slice3/1 -> Register1/1
  Slice4/1 -> Convert2/1
  Convert2/1 -> AddSub/2
  Monostable2/1 -> Counter/1, Delay/1, AddSub/3
  Register1/1 -> SignalLevel/1
  Delay/1 -> Register/3
  Delay1/1 -> Register/2

== system N3Z_tonetest14b/DSProcessor1/OutputRegister/Subsystem ==
  Data : Inport
  PortId : Inport  Port=2
  Write : Inport  Port=3
  Logical : xbsIndex_r4/Logical  logical_function=AND  inputs=2  en=off  latency=0  precision=Full  arith_type=Unsigned  n_bits=8  bin_pt=2  align_bp=on  dbl_ovrd=off  block_type=logical
      settings: xl_area=[1 0 0 1 0 0 0]  block_version=VER_STRING_GOES_HERE
  PortAddress : xbsIndex_r4/Constant  const=0  gui_display_data_type=Fixed-point  arith_type=Unsigned  n_bits=8  bin_pt=0  preci_type=Single  exp_width=8  frac_width=24  explicit_period=on  period=fpgaclk  equ=P=C  opselect=C  inp2=PCIN>>17  opr=+  inp1=P  carry=CIN  dbl_ovrd=off  block_type=constant
      settings: block_version=VER_STRING_GOES_HERE
  Register1 : xbsIndex_r4/Register  init=0  rst=off  en=on  dbl_ovrd=off  block_type=register
      settings: xl_area=[4 8 0 0 0 0 0]  block_version=VER_STRING_GOES_HERE
  Relational1 : xbsIndex_r4/Relational  mode=a=b  op_type=Bool  en=off  latency=0  dbl_ovrd=off  block_type=relational
      settings: xl_area=[2 0 0 4 0 0 0]  block_version=VER_STRING_GOES_HERE
  LatchedData : Outport
  wires:
  Relational1/1 -> Logical/1
  Logical/1 -> Register1/2
  PortAddress/1 -> Relational1/2
  Data/1 -> Register1/1
  PortId/1 -> Relational1/1
  Write/1 -> Logical/2
  Register1/1 -> LatchedData/1

== system N3Z_tonetest14b/DSProcessor1/OutputRegister/Subsystem1 ==
  Data : Inport
  PortId : Inport  Port=2
  Write : Inport  Port=3
  Logical : xbsIndex_r4/Logical  logical_function=AND  inputs=2  en=off  latency=0  precision=Full  arith_type=Unsigned  n_bits=8  bin_pt=2  align_bp=on  dbl_ovrd=off  block_type=logical
      settings: xl_area=[1 0 0 1 0 0 0]  block_version=VER_STRING_GOES_HERE
  PortAddress : xbsIndex_r4/Constant  const=1  gui_display_data_type=Fixed-point  arith_type=Unsigned  n_bits=8  bin_pt=0  preci_type=Single  exp_width=8  frac_width=24  explicit_period=on  period=fpgaclk  equ=P=C  opselect=C  inp2=PCIN>>17  opr=+  inp1=P  carry=CIN  dbl_ovrd=off  block_type=constant
      settings: block_version=VER_STRING_GOES_HERE
  Register1 : xbsIndex_r4/Register  init=0  rst=off  en=on  dbl_ovrd=off  block_type=register
      settings: xl_area=[4 8 0 0 0 0 0]  block_version=VER_STRING_GOES_HERE
  Relational1 : xbsIndex_r4/Relational  mode=a=b  op_type=Bool  en=off  latency=0  dbl_ovrd=off  block_type=relational
      settings: xl_area=[2 0 0 4 0 0 0]  block_version=VER_STRING_GOES_HERE
  LatchedData : Outport
  wires:
  Relational1/1 -> Logical/1
  Logical/1 -> Register1/2
  PortAddress/1 -> Relational1/2
  Data/1 -> Register1/1
  PortId/1 -> Relational1/1
  Write/1 -> Logical/2
  Register1/1 -> LatchedData/1

== system N3Z_tonetest14b/DSProcessor1/OutputRegister/Subsystem10 ==
  Data : Inport
  PortId : Inport  Port=2
  Write : Inport  Port=3
  Logical : xbsIndex_r4/Logical  logical_function=AND  inputs=2  en=off  latency=0  precision=Full  arith_type=Unsigned  n_bits=8  bin_pt=2  align_bp=on  dbl_ovrd=off  block_type=logical
      settings: xl_area=[1 0 0 1 0 0 0]  block_version=VER_STRING_GOES_HERE
  PortAddress : xbsIndex_r4/Constant  const=10  gui_display_data_type=Fixed-point  arith_type=Unsigned  n_bits=8  bin_pt=0  preci_type=Single  exp_width=8  frac_width=24  explicit_period=on  period=fpgaclk  equ=P=C  opselect=C  inp2=PCIN>>17  opr=+  inp1=P  carry=CIN  dbl_ovrd=off  block_type=constant
      settings: block_version=VER_STRING_GOES_HERE
  Register1 : xbsIndex_r4/Register  init=226  rst=off  en=on  dbl_ovrd=off  block_type=register
      settings: xl_area=[4 8 0 0 0 0 0]  block_version=VER_STRING_GOES_HERE
  Relational1 : xbsIndex_r4/Relational  mode=a=b  op_type=Bool  en=off  latency=0  dbl_ovrd=off  block_type=relational
      settings: xl_area=[2 0 0 4 0 0 0]  block_version=VER_STRING_GOES_HERE
  LatchedData : Outport
  wires:
  Relational1/1 -> Logical/1
  Logical/1 -> Register1/2
  PortAddress/1 -> Relational1/2
  Data/1 -> Register1/1
  PortId/1 -> Relational1/1
  Write/1 -> Logical/2
  Register1/1 -> LatchedData/1

== system N3Z_tonetest14b/DSProcessor1/OutputRegister/Subsystem11 ==
  Data : Inport
  PortId : Inport  Port=2
  Write : Inport  Port=3
  Logical : xbsIndex_r4/Logical  logical_function=AND  inputs=2  en=off  latency=0  precision=Full  arith_type=Unsigned  n_bits=8  bin_pt=2  align_bp=on  dbl_ovrd=off  block_type=logical
      settings: xl_area=[1 0 0 1 0 0 0]  block_version=VER_STRING_GOES_HERE
  PortAddress : xbsIndex_r4/Constant  const=11  gui_display_data_type=Fixed-point  arith_type=Unsigned  n_bits=8  bin_pt=0  preci_type=Single  exp_width=8  frac_width=24  explicit_period=on  period=fpgaclk  equ=P=C  opselect=C  inp2=PCIN>>17  opr=+  inp1=P  carry=CIN  dbl_ovrd=off  block_type=constant
      settings: block_version=VER_STRING_GOES_HERE
  Register1 : xbsIndex_r4/Register  init=151  rst=off  en=on  dbl_ovrd=off  block_type=register
      settings: xl_area=[4 8 0 0 0 0 0]  block_version=VER_STRING_GOES_HERE
  Relational1 : xbsIndex_r4/Relational  mode=a=b  op_type=Bool  en=off  latency=0  dbl_ovrd=off  block_type=relational
      settings: xl_area=[2 0 0 4 0 0 0]  block_version=VER_STRING_GOES_HERE
  LatchedData : Outport
  wires:
  Relational1/1 -> Logical/1
  Logical/1 -> Register1/2
  PortAddress/1 -> Relational1/2
  Data/1 -> Register1/1
  PortId/1 -> Relational1/1
  Write/1 -> Logical/2
  Register1/1 -> LatchedData/1

== system N3Z_tonetest14b/DSProcessor1/OutputRegister/Subsystem12 ==
  Data : Inport
  PortId : Inport  Port=2
  Write : Inport  Port=3
  Logical : xbsIndex_r4/Logical  logical_function=AND  inputs=2  en=off  latency=0  precision=Full  arith_type=Unsigned  n_bits=8  bin_pt=2  align_bp=on  dbl_ovrd=off  block_type=logical
      settings: xl_area=[1 0 0 1 0 0 0]  block_version=VER_STRING_GOES_HERE
  PortAddress : xbsIndex_r4/Constant  const=12  gui_display_data_type=Fixed-point  arith_type=Unsigned  n_bits=8  bin_pt=0  preci_type=Single  exp_width=8  frac_width=24  explicit_period=on  period=fpgaclk  equ=P=C  opselect=C  inp2=PCIN>>17  opr=+  inp1=P  carry=CIN  dbl_ovrd=off  block_type=constant
      settings: block_version=VER_STRING_GOES_HERE
  Register1 : xbsIndex_r4/Register  init=151  rst=off  en=on  dbl_ovrd=off  block_type=register
      settings: xl_area=[4 8 0 0 0 0 0]  block_version=VER_STRING_GOES_HERE
  Relational1 : xbsIndex_r4/Relational  mode=a=b  op_type=Bool  en=off  latency=0  dbl_ovrd=off  block_type=relational
      settings: xl_area=[2 0 0 4 0 0 0]  block_version=VER_STRING_GOES_HERE
  LatchedData : Outport
  Ack_Fifo : Outport  Port=2
  wires:
  Relational1/1 -> Logical/1
  Logical/1 -> Register1/2, Ack_Fifo/1
  PortAddress/1 -> Relational1/2
  Data/1 -> Register1/1
  PortId/1 -> Relational1/1
  Write/1 -> Logical/2
  Register1/1 -> LatchedData/1

== system N3Z_tonetest14b/DSProcessor1/OutputRegister/Subsystem13 ==
  Data : Inport
  PortId : Inport  Port=2
  Write : Inport  Port=3
  Logical : xbsIndex_r4/Logical  logical_function=AND  inputs=2  en=off  latency=0  precision=Full  arith_type=Unsigned  n_bits=8  bin_pt=2  align_bp=on  dbl_ovrd=off  block_type=logical
      settings: xl_area=[1 0 0 1 0 0 0]  block_version=VER_STRING_GOES_HERE
  PortAddress : xbsIndex_r4/Constant  const=13  gui_display_data_type=Fixed-point  arith_type=Unsigned  n_bits=8  bin_pt=0  preci_type=Single  exp_width=8  frac_width=24  explicit_period=on  period=fpgaclk  equ=P=C  opselect=C  inp2=PCIN>>17  opr=+  inp1=P  carry=CIN  dbl_ovrd=off  block_type=constant
      settings: block_version=VER_STRING_GOES_HERE
  Register1 : xbsIndex_r4/Register  init=0  rst=off  en=on  dbl_ovrd=off  block_type=register
      settings: xl_area=[4 8 0 0 0 0 0]  block_version=VER_STRING_GOES_HERE
  Relational1 : xbsIndex_r4/Relational  mode=a=b  op_type=Bool  en=off  latency=0  dbl_ovrd=off  block_type=relational
      settings: xl_area=[2 0 0 4 0 0 0]  block_version=VER_STRING_GOES_HERE
  LatchedData : Outport
  NewValue : Outport  Port=2
  wires:
  Relational1/1 -> Logical/1
  Logical/1 -> Register1/2, NewValue/1
  PortAddress/1 -> Relational1/2
  Data/1 -> Register1/1
  PortId/1 -> Relational1/1
  Write/1 -> Logical/2
  Register1/1 -> LatchedData/1

== system N3Z_tonetest14b/DSProcessor1/OutputRegister/Subsystem14 ==
  Data : Inport
  PortId : Inport  Port=2
  Write : Inport  Port=3
  Logical : xbsIndex_r4/Logical  logical_function=AND  inputs=2  en=off  latency=0  precision=Full  arith_type=Unsigned  n_bits=8  bin_pt=2  align_bp=on  dbl_ovrd=off  block_type=logical
      settings: xl_area=[1 0 0 1 0 0 0]  block_version=VER_STRING_GOES_HERE
  PortAddress : xbsIndex_r4/Constant  const=14  gui_display_data_type=Fixed-point  arith_type=Unsigned  n_bits=8  bin_pt=0  preci_type=Single  exp_width=8  frac_width=24  explicit_period=on  period=fpgaclk  equ=P=C  opselect=C  inp2=PCIN>>17  opr=+  inp1=P  carry=CIN  dbl_ovrd=off  block_type=constant
      settings: block_version=VER_STRING_GOES_HERE
  Register1 : xbsIndex_r4/Register  init=0  rst=off  en=on  dbl_ovrd=off  block_type=register
      settings: xl_area=[4 8 0 0 0 0 0]  block_version=VER_STRING_GOES_HERE
  Relational1 : xbsIndex_r4/Relational  mode=a=b  op_type=Bool  en=off  latency=0  dbl_ovrd=off  block_type=relational
      settings: xl_area=[2 0 0 4 0 0 0]  block_version=VER_STRING_GOES_HERE
  LatchedData : Outport
  wires:
  Relational1/1 -> Logical/1
  Logical/1 -> Register1/2
  PortAddress/1 -> Relational1/2
  Data/1 -> Register1/1
  PortId/1 -> Relational1/1
  Write/1 -> Logical/2
  Register1/1 -> LatchedData/1

== system N3Z_tonetest14b/DSProcessor1/OutputRegister/Subsystem15 ==
  Data : Inport
  PortId : Inport  Port=2
  Write : Inport  Port=3
  Logical : xbsIndex_r4/Logical  logical_function=AND  inputs=2  en=off  latency=0  precision=Full  arith_type=Unsigned  n_bits=8  bin_pt=2  align_bp=on  dbl_ovrd=off  block_type=logical
      settings: xl_area=[1 0 0 1 0 0 0]  block_version=VER_STRING_GOES_HERE
  PortAddress : xbsIndex_r4/Constant  const=15  gui_display_data_type=Fixed-point  arith_type=Unsigned  n_bits=8  bin_pt=0  preci_type=Single  exp_width=8  frac_width=24  explicit_period=on  period=fpgaclk  equ=P=C  opselect=C  inp2=PCIN>>17  opr=+  inp1=P  carry=CIN  dbl_ovrd=off  block_type=constant
      settings: block_version=VER_STRING_GOES_HERE
  Register1 : xbsIndex_r4/Register  init=0  rst=off  en=on  dbl_ovrd=off  block_type=register
      settings: xl_area=[4 8 0 0 0 0 0]  block_version=VER_STRING_GOES_HERE
  Relational1 : xbsIndex_r4/Relational  mode=a=b  op_type=Bool  en=off  latency=0  dbl_ovrd=off  block_type=relational
      settings: xl_area=[2 0 0 4 0 0 0]  block_version=VER_STRING_GOES_HERE
  LatchedData : Outport
  wires:
  Relational1/1 -> Logical/1
  Logical/1 -> Register1/2
  PortAddress/1 -> Relational1/2
  Data/1 -> Register1/1
  PortId/1 -> Relational1/1
  Write/1 -> Logical/2
  Register1/1 -> LatchedData/1

== system N3Z_tonetest14b/DSProcessor1/OutputRegister/Subsystem16 ==
  Data : Inport
  PortId : Inport  Port=2
  Write : Inport  Port=3
  Logical : xbsIndex_r4/Logical  logical_function=AND  inputs=2  en=off  latency=0  precision=Full  arith_type=Unsigned  n_bits=8  bin_pt=2  align_bp=on  dbl_ovrd=off  block_type=logical
      settings: xl_area=[1 0 0 1 0 0 0]  block_version=VER_STRING_GOES_HERE
  PortAddress : xbsIndex_r4/Constant  const=16  gui_display_data_type=Fixed-point  arith_type=Unsigned  n_bits=8  bin_pt=0  preci_type=Single  exp_width=8  frac_width=24  explicit_period=on  period=fpgaclk  equ=P=C  opselect=C  inp2=PCIN>>17  opr=+  inp1=P  carry=CIN  dbl_ovrd=off  block_type=constant
      settings: block_version=VER_STRING_GOES_HERE
  Register1 : xbsIndex_r4/Register  init=0  rst=off  en=on  dbl_ovrd=off  block_type=register
      settings: xl_area=[4 8 0 0 0 0 0]  block_version=VER_STRING_GOES_HERE
  Relational1 : xbsIndex_r4/Relational  mode=a=b  op_type=Bool  en=off  latency=0  dbl_ovrd=off  block_type=relational
      settings: xl_area=[2 0 0 4 0 0 0]  block_version=VER_STRING_GOES_HERE
  LatchedData : Outport
  wires:
  Relational1/1 -> Logical/1
  Logical/1 -> Register1/2
  PortAddress/1 -> Relational1/2
  Data/1 -> Register1/1
  PortId/1 -> Relational1/1
  Write/1 -> Logical/2
  Register1/1 -> LatchedData/1

== system N3Z_tonetest14b/DSProcessor1/OutputRegister/Subsystem17 ==
  Data : Inport
  PortId : Inport  Port=2
  Write : Inport  Port=3
  Logical : xbsIndex_r4/Logical  logical_function=AND  inputs=2  en=off  latency=0  precision=Full  arith_type=Unsigned  n_bits=8  bin_pt=2  align_bp=on  dbl_ovrd=off  block_type=logical
      settings: xl_area=[1 0 0 1 0 0 0]  block_version=VER_STRING_GOES_HERE
  PortAddress : xbsIndex_r4/Constant  const=17  gui_display_data_type=Fixed-point  arith_type=Unsigned  n_bits=8  bin_pt=0  preci_type=Single  exp_width=8  frac_width=24  explicit_period=on  period=fpgaclk  equ=P=C  opselect=C  inp2=PCIN>>17  opr=+  inp1=P  carry=CIN  dbl_ovrd=off  block_type=constant
      settings: block_version=VER_STRING_GOES_HERE
  Register1 : xbsIndex_r4/Register  init=1  rst=off  en=on  dbl_ovrd=off  block_type=register
      settings: xl_area=[4 8 0 0 0 0 0]  block_version=VER_STRING_GOES_HERE
  Relational1 : xbsIndex_r4/Relational  mode=a=b  op_type=Bool  en=off  latency=0  dbl_ovrd=off  block_type=relational
      settings: xl_area=[2 0 0 4 0 0 0]  block_version=VER_STRING_GOES_HERE
  LatchedData : Outport
  wires:
  Relational1/1 -> Logical/1
  Logical/1 -> Register1/2
  PortAddress/1 -> Relational1/2
  Data/1 -> Register1/1
  PortId/1 -> Relational1/1
  Write/1 -> Logical/2
  Register1/1 -> LatchedData/1

== system N3Z_tonetest14b/DSProcessor1/OutputRegister/Subsystem18 ==
  Data : Inport
  PortId : Inport  Port=2
  Write : Inport  Port=3
  Logical : xbsIndex_r4/Logical  logical_function=AND  inputs=2  en=off  latency=0  precision=Full  arith_type=Unsigned  n_bits=8  bin_pt=2  align_bp=on  dbl_ovrd=off  block_type=logical
      settings: xl_area=[1 0 0 1 0 0 0]  block_version=VER_STRING_GOES_HERE
  PortAddress : xbsIndex_r4/Constant  const=18  gui_display_data_type=Fixed-point  arith_type=Unsigned  n_bits=8  bin_pt=0  preci_type=Single  exp_width=8  frac_width=24  explicit_period=on  period=fpgaclk  equ=P=C  opselect=C  inp2=PCIN>>17  opr=+  inp1=P  carry=CIN  dbl_ovrd=off  block_type=constant
      settings: block_version=VER_STRING_GOES_HERE
  Register1 : xbsIndex_r4/Register  init=0  rst=off  en=on  dbl_ovrd=off  block_type=register
      settings: xl_area=[4 8 0 0 0 0 0]  block_version=VER_STRING_GOES_HERE
  Relational1 : xbsIndex_r4/Relational  mode=a=b  op_type=Bool  en=off  latency=0  dbl_ovrd=off  block_type=relational
      settings: xl_area=[2 0 0 4 0 0 0]  block_version=VER_STRING_GOES_HERE
  LatchedData : Outport
  wires:
  Relational1/1 -> Logical/1
  Logical/1 -> Register1/2
  PortAddress/1 -> Relational1/2
  Data/1 -> Register1/1
  PortId/1 -> Relational1/1
  Write/1 -> Logical/2
  Register1/1 -> LatchedData/1

== system N3Z_tonetest14b/DSProcessor1/OutputRegister/Subsystem19 ==
  Data : Inport
  PortId : Inport  Port=2
  Write : Inport  Port=3
  Logical : xbsIndex_r4/Logical  logical_function=AND  inputs=2  en=off  latency=0  precision=Full  arith_type=Unsigned  n_bits=8  bin_pt=2  align_bp=on  dbl_ovrd=off  block_type=logical
      settings: xl_area=[1 0 0 1 0 0 0]  block_version=VER_STRING_GOES_HERE
  PortAddress : xbsIndex_r4/Constant  const=19  gui_display_data_type=Fixed-point  arith_type=Unsigned  n_bits=8  bin_pt=0  preci_type=Single  exp_width=8  frac_width=24  explicit_period=on  period=fpgaclk  equ=P=C  opselect=C  inp2=PCIN>>17  opr=+  inp1=P  carry=CIN  dbl_ovrd=off  block_type=constant
      settings: block_version=VER_STRING_GOES_HERE
  Register1 : xbsIndex_r4/Register  init=0  rst=off  en=on  dbl_ovrd=off  block_type=register
      settings: xl_area=[4 8 0 0 0 0 0]  block_version=VER_STRING_GOES_HERE
  Relational1 : xbsIndex_r4/Relational  mode=a=b  op_type=Bool  en=off  latency=0  dbl_ovrd=off  block_type=relational
      settings: xl_area=[2 0 0 4 0 0 0]  block_version=VER_STRING_GOES_HERE
  LatchedData : Outport
  wires:
  Relational1/1 -> Logical/1
  Logical/1 -> Register1/2
  PortAddress/1 -> Relational1/2
  Data/1 -> Register1/1
  PortId/1 -> Relational1/1
  Write/1 -> Logical/2
  Register1/1 -> LatchedData/1
